simulink model "OBC2v1dot"  (R2017a)
settings: Solver=VariableStepAuto  StartTime=0.0  StopTime=10.0  RelTol=1e-3
settings Model: Creator=pc  LastModifiedBy=pc

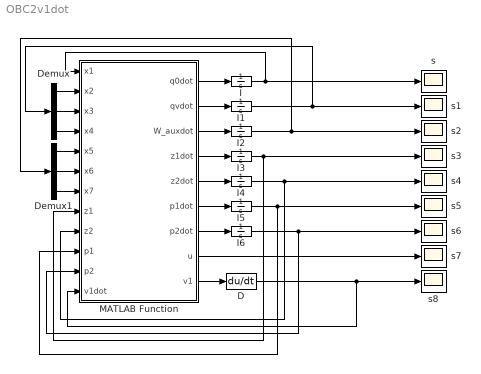
== system OBC2v1dot ==
  D : Derivative
  Demux : Demux  Outputs=3
  Demux1 : Demux  Outputs=3
  I : Integrator  InitialCondition=0.8224
  I1 : Integrator  InitialCondition=[0.2226 0.4397 0.3604]'
  I2 : Integrator  InitialCondition=[-1.5 -5.8 -6.8]'
  I3 : Integrator  InitialCondition=[0.5 0.2 0.3]'
  I4 : Integrator  InitialCondition=[0.5 0.2 0.3]'
  I5 : Integrator  InitialCondition=[1 0 0;0 1 0;0 0 1]
  I6 : Integrator  InitialCondition=[1 0 0;0 1 0;0 0 1]
  MATLAB Function : MATLAB Function  TreatAsAtomicUnit=on
  s{,1..8} (9 alike) : Scope
  wires:
  MATLAB Function/9(v1) -> D/1
  MATLAB Function/1(q0dot) -> I/1
  MATLAB Function/2(qvdot) -> I1/1
  MATLAB Function/3(W_auxdot) -> I2/1
  MATLAB Function/4(z1dot) -> I3/1
  MATLAB Function/5(z2dot) -> I4/1
  I4/1 -> s4/1, MATLAB Function/9(z2)
  MATLAB Function/6(p1dot) -> I5/1
  I5/1 -> MATLAB Function/10(p1), s5/1
  MATLAB Function/7(p2dot) -> I6/1
  I6/1 -> s6/1, MATLAB Function/11(p2)
  Demux/1 -> MATLAB Function/2(x2)
  Demux/2 -> MATLAB Function/3(x3)
  Demux/3 -> MATLAB Function/4(x4)
  I/1 -> s/1, MATLAB Function/1(x1)
  I1/1 -> s1/1, Demux/1
  Demux1/2 -> MATLAB Function/6(x6)
  Demux1/3 -> MATLAB Function/7(x7)
  Demux1/1 -> MATLAB Function/5(x5)
  I2/1 -> s2/1, Demux1/1
  I3/1 -> MATLAB Function/8(z1), s3/1
  MATLAB Function/8(u) -> s7/1
  D/1 -> MATLAB Function/12(v1dot), s8/1

== matlab function OBC2v1dot/MATLAB Function ==
  data: x1 input; x2 input; x3 input; x4 input; x5 input; x6 input; x7 input; q0dot output; qvdot output; W_auxdot output; z1dot output; z2dot output; p1dot output; p2dot output; u output; v1 output; z1 input; z2 input; p1 input; p2 input; v1dot input
function [q0dot,qvdot,W_auxdot,z1dot,z2dot,p1dot,p2dot,u,v1] = fctt(x1,x2,x3,x4,x5,x6,x7,z1,z2,p1,p2,v1dot)
Q0=0.8224;
R1=0.1*eye(3,3);
v=[0.0098,0.0098,0.0176];
J=diag(v);
%R2=0.03*eye(3,3);
IR2=33.3333*eye(3,3);
gamma= 150;
Q1=eye(3,3);
Q2=eye(3,3);
B2=102.0408*eye(3,3);%equation(20)
G2=102.0408*eye(3,3);
B22=102.0408*eye(3,3);
W_d=[0;0;0];
%--------------------------------------------------------------------------------------------------------------------
R_T=[ x1^2+x2^2-x3^2-x4^2, 2*(x2*x3+x1*x4), 2*(x2*x4-x1*x3)   
          2*(x2*x3-x1*x4), x1^2-x2^2+x3^2-x4^2, 2*(x3*x4+x1*x2)   
          2*(x2*x4+x1*x3), 2*(x3*x4-x1*x2), x1^2-x2^2-x3^2+x4^2];%equation(9)
W_star=R_T*W_d;
q0=x1;
qv=[x2;x3;x4];
W_aux=[x5;x6;x7];
W=W_aux+W_star;
S_T_W=-[0,-W(3),W(2);W(3),0,-W(1);-W(2),W(1),0];
%--------------------------------------------------------------------------------------------------------------------
B1=0.5*[0,-x4,x3;x4,0,-x2;-x3,x2,0]+q0*eye(3,3);%equation(26.2)
A2=(-B2*[0,-x7,x6;x7,0,-x5;-x6,x5,0]*J-B2*[0,-W_star(3),W_star(2);W_star(3),0,-W_star(1);-W_star(2),W_star(1),0]*J);%equation(20)
%--------------------------------------------------------------------------------------------------------------------
v1=-inv(R1)*B1'*p1*qv*sign(Q0)+[0;0;0];%equation(84)
Psi2=-IR2*B2'*p2*z2;
W2=1/(2*gamma^2)*B22'*p2*z2;%equation(88)
q0dot=-0.5*qv'*v1*sign(Q0);%equation(21)
qvdot=B1*v1*sign(Q0);
z1dot=B1*z2-B1*R1\B1'*p1*z1;
z2dot=A2*z2+B2*Psi2-p2\B1'*p1*z1;
p1dot=p1*B1*R1\B1'*p1-Q1;%equation(97)
v2=IR2*B2'*p2*z2+J*v1dot*sign(Q0)-J*A2*v1*sign(Q0)+J*p2\B1'*p1*z1-J*B22*W2;
W_auxdot=A2*W_aux+B2*v2+B22*W2;%equation(26.2)
p1dot=p1dot(:);
T2=1/(2*gamma^2)*G2*(G2')-B2*IR2*B2';%equation(98)
p2dot=-A2.'*p2-p2*A2-p2*T2*p2-Q2;%equation(98)
p2dot=p2dot(:);
u=v2+[0,-x7,x6;x7,0,-x5;-x6,x5,0]*J*W_star+[0,-W_star(3),W_star(2);W_star(3),0,-W_star(1);-W_star(2),W_star(1),0]*J*W_star+J*S_T_W*W_star;
end
